simulink model "Movement"  (R2015a)
settings: Solver=ode3  StartTime=0.0  StopTime=10  FixedStep=0.01  RelTol=1e-3
settings Model: Creator=Nick  LastModifiedBy=Nick

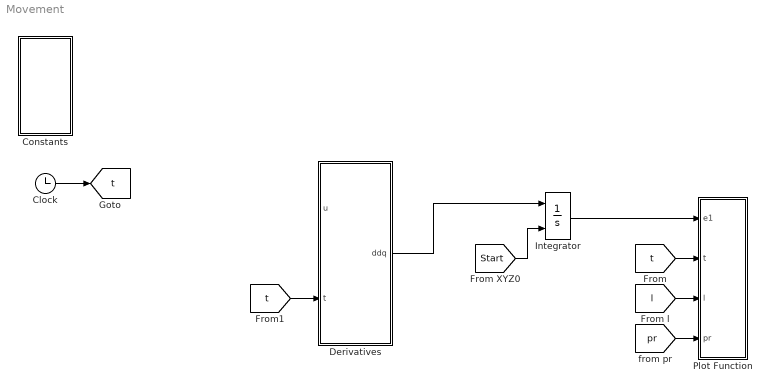
== system Movement ==
  Clock : Clock
  Constants : Subsystem
  Derivatives : MATLAB Function  TreatAsAtomicUnit=on
  Integrator : Integrator  InitialConditionSource=external  ContinuousStateAttributes='Velocity'
  Plot Function : MATLAB Function  TreatAsAtomicUnit=on
  tag scope: t=global
  wires:
  Derivatives/1(ddq) -> Integrator/1
  Integrator/1 -> Plot Function/1(e1)
  [Start] -> Integrator/2
  [l] -> Plot Function/3(l)
  [pr] -> Plot Function/4(pr)
  Clock/1 -> [t]
  [t] -> Plot Function/2(t)
  [t] -> Derivatives/2(t)

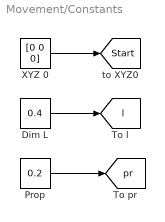
== system Movement/Constants ==
  Dim L : Constant  Value=0.4
  Prop : Constant  Value=0.2
  XYZ 0 : Constant  Value=[0 0 0]
  tag scope: Start=global, l=global, pr=global
  wires:
  XYZ 0/1 -> [Start]
  Dim L/1 -> [l]
  Prop/1 -> [pr]

== matlab function Movement/Derivatives ==
  data: u input; t input; ddq output
function ddq  = Dynamics(u,t) %#ok<*INUSD>
%%control action
dummy = u + 1; % None implemented yet, just included for completeness 
%%Accelerations in Inertial Frame
ddx = 0.3; %Acc in X
ddy = 0.5; %Acc in Y
ddz = 0.4; %Acc in Z

%%Construct Output Vector
ddq = zeros(3,1);
ddq(1)=ddx;
ddq(2)=ddy;
ddq(3)=ddz;
%Integrals take place outside dynamics function
end

== matlab function Movement/Plot Function ==
  data: e1 input; t input; l input; pr input
function plot(e1,t,l,pr)
%Input t
X = e1(1);
Y = e1(2);
Z = e1(3);
%Calculate Motor Positions
mtr1 = ([X+l Y Z]);
mtr2 = ([X Y+l Z]);
mtr3 = ([X-l Y Z]);
mtr4 = ([X Y-l Z]);
%%Calculate Body Attidue

%%Calculate Motor Attitudes

%%Open Figure if first time instance
if(t==0);
    fig = figure();
    hold on;
    grid on;
end
%%Clear and Construct Figure
hold off;
clf();
xlim([-1 5]);
ylim([-1 5]);
zlim([0 3]);
view([4 4 3]);
grid on;
hold on;
%%Display Time
%disp(t);
%%Plot Quad Function
plotCircle3D([X Y 0],[0 0 1],(l),'black');
plot3(([mtr1(1) mtr3(1)]),([mtr1(2) mtr3(2)]),([mtr1(3) mtr3(3)]),'LineWidth',1,'Color','Blue');
plot3(([mtr2(1) mtr4(1)]),([mtr2(2) mtr4(2)]),([mtr2(3) mtr4(3)]),'LineWidth',1,'Color','Blue');
plotCircle3D(mtr1,[0 0 1],pr,'red');
plotCircle3D(mtr2,[0 0 1],pr,'red');
plotCircle3D(mtr3,[0 0 1],pr,'red');
plotCircle3D(mtr4,[0 0 1],pr,'red');
plotCircle3D([X Y Z],[0 0 1],(l+pr),'green');
%%
end
